simulink model "ssp_trigger"  (Simulink 7.3)
settings: Solver=VariableStepDiscrete  StartTime=0.0  StopTime=10.0  RelTol=1e-3
libraries: xbsIndex_r4 x9, nort_sysgenlib x1
settings Model: Creator=nort  LastModifiedBy=nort
settings OptimizationCC: InitFltsAndDblsToZero=on
settings DebuggingCC: SaveWithParameterizedLinksMsg=none  SignalResolutionControl=TryResolveAllWithWarning
settings GRTTargetCC: TargetFcnLib=ansi_tfl_tmw.mat

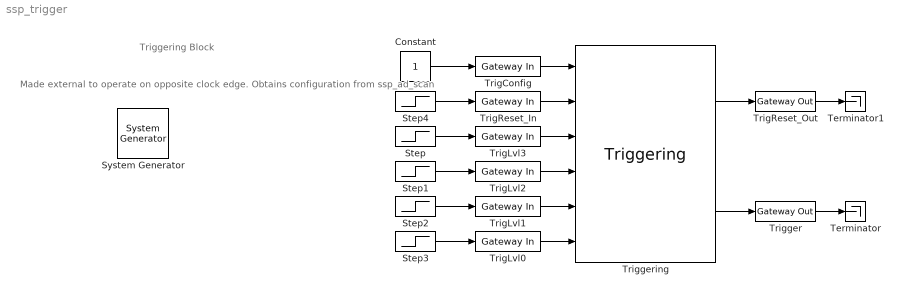
== system ssp_trigger ==
  note: Triggering Block
  note: Made external to operate on opposite clock edge.
      | Obtains configuration from ssp_ad_scan
  " System Generator" : xbsIndex_r4/ System Generator  Tag=genX  SystemSampleTime=-1  xilinxfamily=virtex4  part=xc4vlx25  speed=-10  package=ff668  synthesis_tool=XST  clock_wrapper=Clock Enables  directory=./net_trigger  testbench=off  simulink_period=1  sysclk_period=10  dcm_input_clock_period=10  incr_netlist=off  trim_vbits=Everywhere in SubSystem  dbl_ovrd=According to Block Masks  core_generation=According to Block Masks  run_coregen=off  deprecated_control=off  eval_field=0  block_type=sysgen
      settings: block_version=8.2
  Constant : Constant  OutDataType=sfix(16)  OutScaling=2^0
  Step{,1..4} (5 alike) : Step  Time=5  SampleTime=0
  Terminator : Terminator
  Terminator1 : Terminator
  TrigConfig : xbsIndex_r4/Gateway In  arith_type=Unsigned  n_bits=4  bin_pt=0  quantization="Round  (unbiased: +/- Inf)"  overflow=Saturate  period=1  dbl_ovrd=off  timing_constraint=None  locs_specified=off  LOCs={}  hdl_port=on  block_type=gatewayin
      settings: infoedit="Gateway in block.  Converts inputs of type Simulink integer, double and fixed point to  Xilinx fixed point type.<P><P>Hardware notes:  In hardware these blocks become top level input ports."  block_version=9.2.01
  TrigLvl{0..3} (4 alike) : xbsIndex_r4/Gateway In  arith_type=Boolean  n_bits=16  bin_pt=14  quantization="Round  (unbiased: +/- Inf)"  overflow=Saturate  period=1  dbl_ovrd=off  timing_constraint=None  locs_specified=off  LOCs={}  hdl_port=on  block_type=gatewayin
      settings: infoedit="Gateway in block.  Converts inputs of type Simulink integer, double and fixed point to  Xilinx fixed point type.<P><P>Hardware notes:  In hardware these blocks become top level input ports."  block_version=9.2.01
  TrigReset_In : xbsIndex_r4/Gateway In  arith_type=Boolean  n_bits=1  bin_pt=0  quantization="Round  (unbiased: +/- Inf)"  overflow=Saturate  period=1  dbl_ovrd=off  timing_constraint=None  locs_specified=off  LOCs={}  hdl_port=on  block_type=gatewayin
      settings: infoedit="Gateway in block.  Converts inputs of type Simulink integer, double and fixed point to  Xilinx fixed point type.<P><P>Hardware notes:  In hardware these blocks become top level input ports."  block_version=9.2.01
  TrigReset_Out : xbsIndex_r4/Gateway Out  hdl_port=on  timing_constraint=None  locs_specified=off  LOCs={}  block_type=gatewayout
      settings: infoedit="Gateway out block.  Converts Xilinx fixed point inputs into ouputs of type Simulink integer, double, or fixed point.<P><P>Hardware notes:  In hardware these blocks become top level output ports or are discarded, depending on how they are configured."  block_version=9.2.01
  Trigger : xbsIndex_r4/Gateway Out  hdl_port=on  timing_constraint=None  locs_specified=off  LOCs={}  block_type=gatewayout
      settings: infoedit="Gateway out block.  Converts Xilinx fixed point inputs into ouputs of type Simulink integer, double, or fixed point.<P><P>Hardware notes:  In hardware these blocks become top level output ports or are discarded, depending on how they are configured."  block_version=9.2.01
  Triggering : nort_sysgenlib/Triggering  SystemSampleTime=-1
  wires:
  Step/1 -> TrigLvl3/1
  Step1/1 -> TrigLvl2/1
  Step2/1 -> TrigLvl1/1
  Step3/1 -> TrigLvl0/1
  Constant/1 -> TrigConfig/1
  Trigger/1 -> Terminator/1
  Step4/1 -> TrigReset_In/1
  Triggering/2 -> Trigger/1
  TrigReset_Out/1 -> Terminator1/1
  Triggering/1 -> TrigReset_Out/1
  TrigConfig/1 -> Triggering/1
  TrigReset_In/1 -> Triggering/2
  TrigLvl3/1 -> Triggering/3
  TrigLvl2/1 -> Triggering/4
  TrigLvl1/1 -> Triggering/5
  TrigLvl0/1 -> Triggering/6
